simulink library "LIB_UserCommand"  (R2018b)
settings: Solver=VariableStepAuto  StartTime=0.0  StopTime=10.0  RelTol=1e-3
undefined symbols (not defined in the file or in its folder): NCyclePerMinIncrement, pBlowerValveOutletStaticTgtIncrement, pPatientValveInletTgtIncrement, rInhalationPerCycleDefault
libraries: RespiratorCtrlLib x15
settings Model: Creator=BRAUL  LastModifiedBy=BRAUL

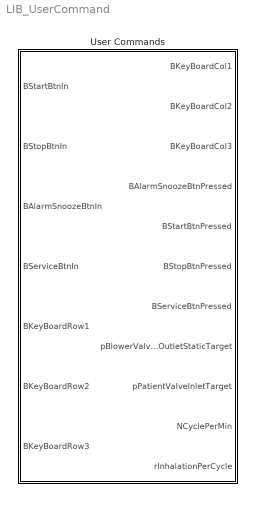
== system LIB_UserCommand ==
  User Commands : Subsystem
      settings: AttributesFormatString=%<ReferenceBlock>

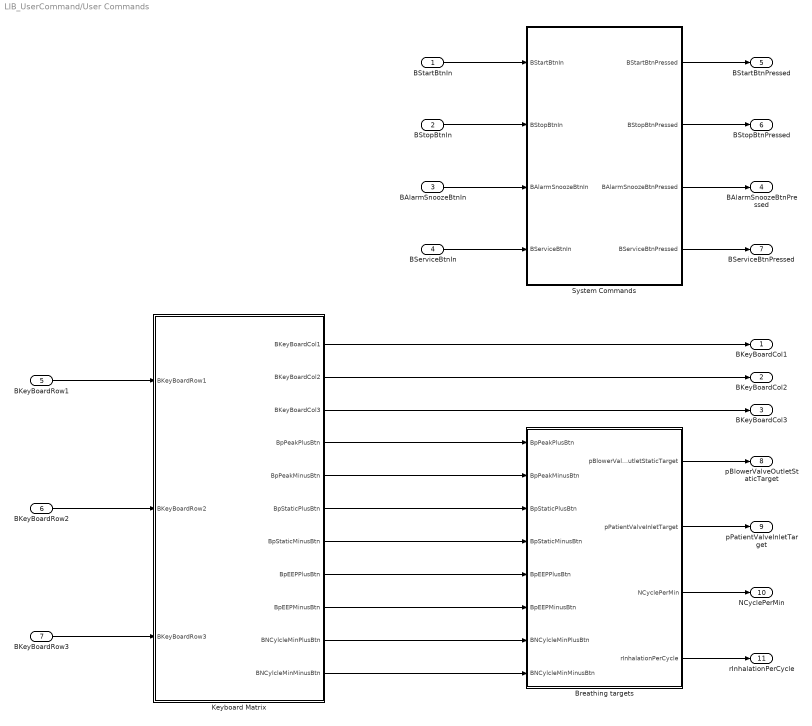
== system LIB_UserCommand/User Commands ==
  BStartBtnIn : Inport  OutDataTypeStr=boolean
  BStopBtnIn : Inport  Port=2  OutDataTypeStr=boolean
  BAlarmSnoozeBtnIn : Inport  Port=3  OutDataTypeStr=boolean
  BServiceBtnIn : Inport  Port=4  OutDataTypeStr=boolean
  BKeyBoardRow1 : Inport  Port=5  OutDataTypeStr=boolean  PortDimensions=1
  BKeyBoardRow2 : Inport  Port=6  OutDataTypeStr=boolean  PortDimensions=1
  BKeyBoardRow3 : Inport  Port=7  OutDataTypeStr=boolean  PortDimensions=1
  Breathing targets : Subsystem
  Keyboard Matrix : Subsystem
  System Commands : Subsystem
  BKeyBoardCol1 : Outport  OutDataTypeStr=boolean  PortDimensions=1
  BKeyBoardCol2 : Outport  Port=2  OutDataTypeStr=boolean  PortDimensions=1
  BKeyBoardCol3 : Outport  Port=3  OutDataTypeStr=boolean  PortDimensions=1
  BAlarmSnoozeBtnPressed : Outport  Port=4  OutDataTypeStr=boolean
  BStartBtnPressed : Outport  Port=5  OutDataTypeStr=boolean
  BStopBtnPressed : Outport  Port=6  OutDataTypeStr=boolean
  BServiceBtnPressed : Outport  Port=7  OutDataTypeStr=boolean
  pBlowerValveOutletStaticTarget : Outport  Port=8
  pPatientValveInletTarget : Outport  Port=9
  NCyclePerMin : Outport  Port=10
  rInhalationPerCycle : Outport  Port=11
  wires:
  BKeyBoardRow3/1 -> Keyboard Matrix/3(BKeyBoardRow3)
  BKeyBoardRow2/1 -> Keyboard Matrix/2(BKeyBoardRow2)
  BKeyBoardRow1/1 -> Keyboard Matrix/1(BKeyBoardRow1)
  Keyboard Matrix/3(BKeyBoardCol3) -> BKeyBoardCol3/1
  Keyboard Matrix/2(BKeyBoardCol2) -> BKeyBoardCol2/1
  Keyboard Matrix/1(BKeyBoardCol1) -> BKeyBoardCol1/1
  Keyboard Matrix/4(BpPeakPlusBtn) -> Breathing targets/1(BpPeakPlusBtn)
  Keyboard Matrix/5(BpPeakMinusBtn) -> Breathing targets/2(BpPeakMinusBtn)
  Keyboard Matrix/6(BpStaticPlusBtn) -> Breathing targets/3(BpStaticPlusBtn)
  Keyboard Matrix/7(BpStaticMinusBtn) -> Breathing targets/4(BpStaticMinusBtn)
  Keyboard Matrix/8(BpEEPPlusBtn) -> Breathing targets/5(BpEEPPlusBtn)
  Keyboard Matrix/9(BpEEPMinusBtn) -> Breathing targets/6(BpEEPMinusBtn)
  Keyboard Matrix/10(BNCylcleMinPlusBtn) -> Breathing targets/7(BNCylcleMinPlusBtn)
  Keyboard Matrix/11(BNCylcleMinMinusBtn) -> Breathing targets/8(BNCylcleMinMinusBtn)
  BStartBtnIn/1 -> System Commands/1(BStartBtnIn)
  BStopBtnIn/1 -> System Commands/2(BStopBtnIn)
  BAlarmSnoozeBtnIn/1 -> System Commands/3(BAlarmSnoozeBtnIn)
  BServiceBtnIn/1 -> System Commands/4(BServiceBtnIn)
  System Commands/1(BStartBtnPressed) -> BStartBtnPressed/1
  System Commands/2(BStopBtnPressed) -> BStopBtnPressed/1
  System Commands/3(BAlarmSnoozeBtnPressed) -> BAlarmSnoozeBtnPressed/1
  System Commands/4(BServiceBtnPressed) -> BServiceBtnPressed/1
  Breathing targets/1(pBlowerValveOutletStaticTarget) -> pBlowerValveOutletStaticTarget/1
  Breathing targets/2(pPatientValveInletTarget) -> pPatientValveInletTarget/1
  Breathing targets/3(NCyclePerMin) -> NCyclePerMin/1
  Breathing targets/4(rInhalationPerCycle) -> rInhalationPerCycle/1

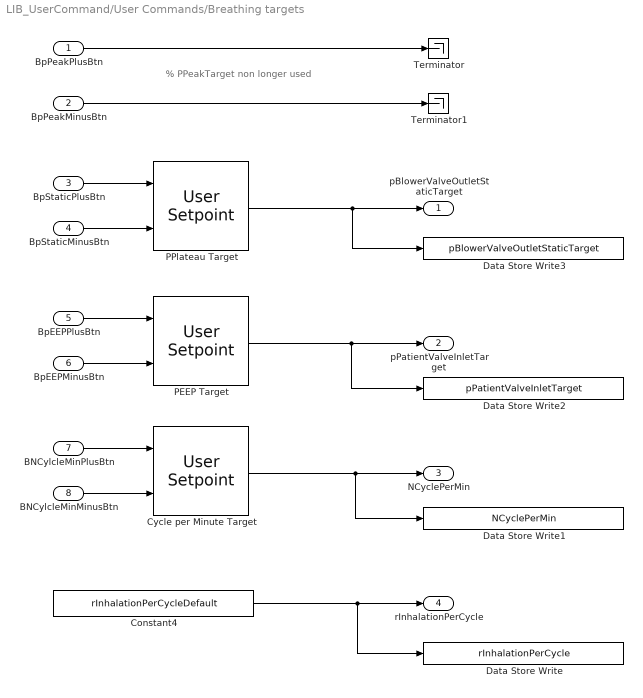
== system LIB_UserCommand/User Commands/Breathing targets ==
  note: % PPeakTarget non longer used
  BpPeakPlusBtn : Inport  OutDataTypeStr=boolean  PortDimensions=1
  BpPeakMinusBtn : Inport  Port=2  OutDataTypeStr=boolean  PortDimensions=1
  BpStaticPlusBtn : Inport  Port=3  OutDataTypeStr=boolean  PortDimensions=1
  BpStaticMinusBtn : Inport  Port=4  OutDataTypeStr=boolean  PortDimensions=1
  BpEEPPlusBtn : Inport  Port=5  OutDataTypeStr=boolean  PortDimensions=1
  BpEEPMinusBtn : Inport  Port=6  OutDataTypeStr=boolean  PortDimensions=1
  BNCylcleMinPlusBtn : Inport  Port=7  OutDataTypeStr=boolean  PortDimensions=1
  BNCylcleMinMinusBtn : Inport  Port=8  OutDataTypeStr=boolean  PortDimensions=1
  Constant4 : Constant  Value=rInhalationPerCycleDefault
  Cycle per Minute Target : RespiratorCtrlLib/Inputs/User Setpoint  DefaultSetPoint=NCyclePerMinDefault  Increment=NCyclePerMinIncrement  Decrement=NCyclePerMinDecrement  MinSetPoint=NCyclePerMinMin  MaxSetPoint=NCyclePerMinMax
  Data Store Write : DataStoreWrite  DataStoreName=rInhalationPerCycle
  Data Store Write1 : DataStoreWrite  DataStoreName=NCyclePerMin
  Data Store Write2 : DataStoreWrite  DataStoreName=pPatientValveInletTarget
  Data Store Write3 : DataStoreWrite  DataStoreName=pBlowerValveOutletStaticTarget
  PEEP Target : RespiratorCtrlLib/Inputs/User Setpoint  DefaultSetPoint=pPatientValveInletTgtDefault  Increment=pPatientValveInletTgtIncrement  Decrement=pPatientValveInletTgtDecrement  MinSetPoint=pPatientValveInletTgtMin  MaxSetPoint=pPatientValveInletTgtMax
  PPlateau Target : RespiratorCtrlLib/Inputs/User Setpoint  DefaultSetPoint=pBlowerValveOutletStaticTgtDefault  Increment=pBlowerValveOutletStaticTgtIncrement  Decrement=pBlowerValveOutletStaticTgtDecrement  MinSetPoint=pBlowerValveOutletStaticTgtMin  MaxSetPoint=pBlowerValveOutletStaticTgtMax
  Terminator : Terminator
  Terminator1 : Terminator
  pBlowerValveOutletStaticTarget : Outport
  pPatientValveInletTarget : Outport  Port=2
  NCyclePerMin : Outport  Port=3
  rInhalationPerCycle : Outport  Port=4
  wires:
  BpPeakMinusBtn/1 -> Terminator1/1
  BpPeakPlusBtn/1 -> Terminator/1
  BNCylcleMinMinusBtn/1 -> Cycle per Minute Target/2
  BNCylcleMinPlusBtn/1 -> Cycle per Minute Target/1
  BpEEPMinusBtn/1 -> PEEP Target/2
  BpEEPPlusBtn/1 -> PEEP Target/1
  BpStaticMinusBtn/1 -> PPlateau Target/2
  BpStaticPlusBtn/1 -> PPlateau Target/1
  Constant4/1 -> rInhalationPerCycle/1, Data Store Write/1
  PEEP Target/1 -> pPatientValveInletTarget/1, Data Store Write2/1
  PPlateau Target/1 -> Data Store Write3/1, pBlowerValveOutletStaticTarget/1
  Cycle per Minute Target/1 -> NCyclePerMin/1, Data Store Write1/1

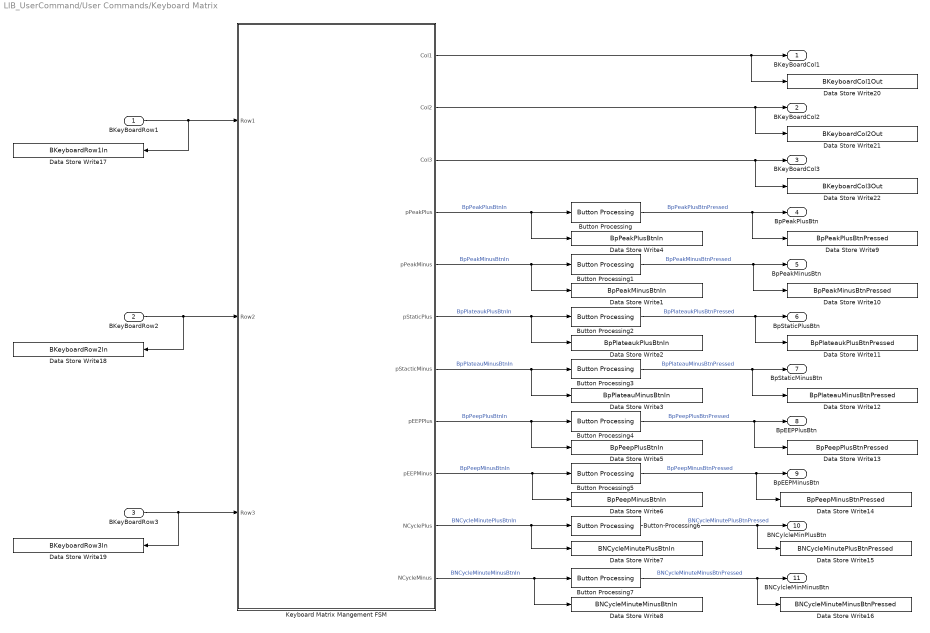
== system LIB_UserCommand/User Commands/Keyboard Matrix ==
  BKeyBoardRow1 : Inport  OutDataTypeStr=boolean  PortDimensions=1
  BKeyBoardRow2 : Inport  Port=2  OutDataTypeStr=boolean  PortDimensions=1
  BKeyBoardRow3 : Inport  Port=3  OutDataTypeStr=boolean  PortDimensions=1
  Button Processing{,1..7} (8 alike) : RespiratorCtrlLib/Inputs/Button Processing  tDebounce=tKeyboardBtnDebounce  tSample=MdlTS
  Data Store Write1 : DataStoreWrite  DataStoreName=BpPeakMinusBtnIn
  Data Store Write10 : DataStoreWrite  DataStoreName=BpPeakMinusBtnPressed
  Data Store Write11 : DataStoreWrite  DataStoreName=BpPlateaukPlusBtnPressed
  Data Store Write12 : DataStoreWrite  DataStoreName=BpPlateauMinusBtnPressed
  Data Store Write13 : DataStoreWrite  DataStoreName=BpPeepPlusBtnPressed
  Data Store Write14 : DataStoreWrite  DataStoreName=BpPeepMinusBtnPressed
  Data Store Write15 : DataStoreWrite  DataStoreName=BNCycleMinutePlusBtnPressed
  Data Store Write16 : DataStoreWrite  DataStoreName=BNCycleMinuteMinusBtnPressed
  Data Store Write17 : DataStoreWrite  DataStoreName=BKeyboardRow1In
  Data Store Write18 : DataStoreWrite  DataStoreName=BKeyboardRow2In
  Data Store Write19 : DataStoreWrite  DataStoreName=BKeyboardRow3In
  Data Store Write2 : DataStoreWrite  DataStoreName=BpPlateaukPlusBtnIn
  Data Store Write20 : DataStoreWrite  DataStoreName=BKeyboardCol1Out
  Data Store Write21 : DataStoreWrite  DataStoreName=BKeyboardCol2Out
  Data Store Write22 : DataStoreWrite  DataStoreName=BKeyboardCol3Out
  Data Store Write3 : DataStoreWrite  DataStoreName=BpPlateauMinusBtnIn
  Data Store Write4 : DataStoreWrite  DataStoreName=BpPeakPlusBtnIn
  Data Store Write5 : DataStoreWrite  DataStoreName=BpPeepPlusBtnIn
  Data Store Write6 : DataStoreWrite  DataStoreName=BpPeepMinusBtnIn
  Data Store Write7 : DataStoreWrite  DataStoreName=BNCycleMinutePlusBtnIn
  Data Store Write8 : DataStoreWrite  DataStoreName=BNCycleMinuteMinusBtnIn
  Data Store Write9 : DataStoreWrite  DataStoreName=BpPeakPlusBtnPressed
  Keyboard Matrix Mangement FSM : Stateflow chart  TreatAsAtomicUnit=on
  BKeyBoardCol1 : Outport  OutDataTypeStr=boolean  PortDimensions=1
  BKeyBoardCol2 : Outport  Port=2  OutDataTypeStr=boolean  PortDimensions=1
  BKeyBoardCol3 : Outport  Port=3  OutDataTypeStr=boolean  PortDimensions=1
  BpPeakPlusBtn : Outport  Port=4  OutDataTypeStr=boolean  PortDimensions=1
  BpPeakMinusBtn : Outport  Port=5  OutDataTypeStr=boolean  PortDimensions=1
  BpStaticPlusBtn : Outport  Port=6  OutDataTypeStr=boolean  PortDimensions=1
  BpStaticMinusBtn : Outport  Port=7  OutDataTypeStr=boolean  PortDimensions=1
  BpEEPPlusBtn : Outport  Port=8  OutDataTypeStr=boolean  PortDimensions=1
  BpEEPMinusBtn : Outport  Port=9  OutDataTypeStr=boolean  PortDimensions=1
  BNCylcleMinPlusBtn : Outport  Port=10  OutDataTypeStr=boolean  PortDimensions=1
  BNCylcleMinMinusBtn : Outport  Port=11  OutDataTypeStr=boolean  PortDimensions=1
  wires:
  Button Processing7/1 -> BNCylcleMinMinusBtn/1, Data Store Write16/1  "BNCycleMinuteMinusBtnPressed"
  Button Processing6/1 -> BNCylcleMinPlusBtn/1, Data Store Write15/1  "BNCycleMinutePlusBtnPressed"
  Button Processing5/1 -> BpEEPMinusBtn/1, Data Store Write14/1  "BpPeepMinusBtnPressed"
  Button Processing4/1 -> BpEEPPlusBtn/1, Data Store Write13/1  "BpPeepPlusBtnPressed"
  Button Processing3/1 -> BpStaticMinusBtn/1, Data Store Write12/1  "BpPlateauMinusBtnPressed"
  Button Processing2/1 -> BpStaticPlusBtn/1, Data Store Write11/1  "BpPlateaukPlusBtnPressed"
  Button Processing1/1 -> BpPeakMinusBtn/1, Data Store Write10/1  "BpPeakMinusBtnPressed"
  Button Processing/1 -> BpPeakPlusBtn/1, Data Store Write9/1  "BpPeakPlusBtnPressed"
  Keyboard Matrix Mangement FSM/10(NCyclePlus) -> Button Processing6/1, Data Store Write7/1  "BNCycleMinutePlusBtnIn"
  Keyboard Matrix Mangement FSM/11(NCycleMinus) -> Button Processing7/1, Data Store Write8/1  "BNCycleMinuteMinusBtnIn"
  Keyboard Matrix Mangement FSM/9(pEEPMinus) -> Button Processing5/1, Data Store Write6/1  "BpPeepMinusBtnIn"
  Keyboard Matrix Mangement FSM/8(pEEPPlus) -> Button Processing4/1, Data Store Write5/1  "BpPeepPlusBtnIn"
  Keyboard Matrix Mangement FSM/7(pStacticMinus) -> Button Processing3/1, Data Store Write3/1  "BpPlateauMinusBtnIn"
  Keyboard Matrix Mangement FSM/6(pStaticPlus) -> Button Processing2/1, Data Store Write2/1  "BpPlateaukPlusBtnIn"
  Keyboard Matrix Mangement FSM/5(pPeakMinus) -> Button Processing1/1, Data Store Write1/1  "BpPeakMinusBtnIn"
  Keyboard Matrix Mangement FSM/4(pPeakPlus) -> Button Processing/1, Data Store Write4/1  "BpPeakPlusBtnIn"
  BKeyBoardRow1/1 -> Keyboard Matrix Mangement FSM/1(Row1), Data Store Write17/1
  BKeyBoardRow2/1 -> Keyboard Matrix Mangement FSM/2(Row2), Data Store Write18/1
  BKeyBoardRow3/1 -> Keyboard Matrix Mangement FSM/3(Row3), Data Store Write19/1
  Keyboard Matrix Mangement FSM/3(Col3) -> BKeyBoardCol3/1, Data Store Write22/1
  Keyboard Matrix Mangement FSM/2(Col2) -> BKeyBoardCol2/1, Data Store Write21/1
  Keyboard Matrix Mangement FSM/1(Col1) -> BKeyBoardCol1/1, Data Store Write20/1

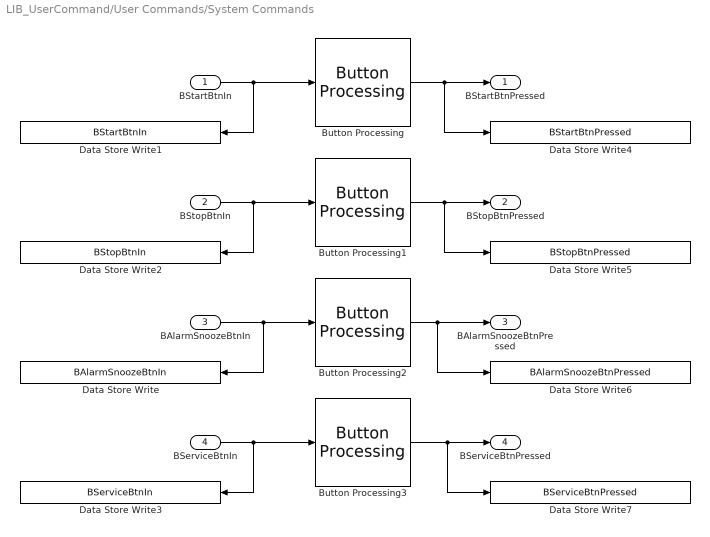
== system LIB_UserCommand/User Commands/System Commands ==
  BStartBtnIn : Inport  OutDataTypeStr=boolean
  BStopBtnIn : Inport  Port=2  OutDataTypeStr=boolean
  BAlarmSnoozeBtnIn : Inport  Port=3  OutDataTypeStr=boolean
  BServiceBtnIn : Inport  Port=4  OutDataTypeStr=boolean
  Button Processing{,1..3} (4 alike) : RespiratorCtrlLib/Inputs/Button Processing  tDebounce=tSystemBtnDebounce  tSample=MdlTS
  Data Store Write : DataStoreWrite  DataStoreName=BAlarmSnoozeBtnIn
  Data Store Write1 : DataStoreWrite  DataStoreName=BStartBtnIn
  Data Store Write2 : DataStoreWrite  DataStoreName=BStopBtnIn
  Data Store Write3 : DataStoreWrite  DataStoreName=BServiceBtnIn
  Data Store Write4 : DataStoreWrite  DataStoreName=BStartBtnPressed
  Data Store Write5 : DataStoreWrite  DataStoreName=BStopBtnPressed
  Data Store Write6 : DataStoreWrite  DataStoreName=BAlarmSnoozeBtnPressed
  Data Store Write7 : DataStoreWrite  DataStoreName=BServiceBtnPressed
  BStartBtnPressed : Outport  OutDataTypeStr=boolean
  BStopBtnPressed : Outport  Port=2  OutDataTypeStr=boolean
  BAlarmSnoozeBtnPressed : Outport  Port=3  OutDataTypeStr=boolean
  BServiceBtnPressed : Outport  Port=4  OutDataTypeStr=boolean
  wires:
  Button Processing/1 -> Data Store Write4/1, BStartBtnPressed/1
  BStartBtnIn/1 -> Data Store Write1/1, Button Processing/1
  BStopBtnIn/1 -> Data Store Write2/1, Button Processing1/1
  BAlarmSnoozeBtnIn/1 -> Data Store Write/1, Button Processing2/1
  BServiceBtnIn/1 -> Data Store Write3/1, Button Processing3/1
  Button Processing1/1 -> Data Store Write5/1, BStopBtnPressed/1
  Button Processing2/1 -> Data Store Write6/1, BAlarmSnoozeBtnPressed/1
  Button Processing3/1 -> Data Store Write7/1, BServiceBtnPressed/1

== stateflow chart LIB_UserCommand/User Commands/Keyboard Matrix/Keyboard Matrix Mangement FSM ==
  state Init
    entry:
    Col1 = true;
    Col2 = false;
    Col3 = false;
  state READ_COL_1
    entry:
    Col1 = false;
    Col2 = true;
    Col3 = false;
    pPeakPlus = Row1;
    pPeakMinus  = Row2;
    pStaticPlus  = Row3;
  state READ_COL_3
    entry:
    Col1 = true;
    Col2 = false;
    Col3 = false;
    NCyclePlus = Row1;
    NCycleMinus  = Row2;
  state READ_COL_2
    entry:
    Col1 = false;
    Col2 = false;
    Col3 = true;
    pStacticMinus = Row1;
    pEEPPlus  = Row2;
    pEEPMinus  = Row3;
  (default) -> Init
  Init -> READ_COL_1
  READ_COL_3 -> READ_COL_1
  READ_COL_1 -> READ_COL_2
  READ_COL_2 -> READ_COL_3
  data: Row1 input boolean; Row2 input boolean; Row3 input boolean; Col1 output boolean =false; Col2 output boolean =false; Col3 output boolean =false; pPeakPlus output boolean =false; pPeakMinus output boolean =false; pStaticPlus output boolean =false; pStacticMinus output boolean =false; pEEPPlus output boolean =false; pEEPMinus output boolean =false; NCyclePlus output boolean =false; NCycleMinus output boolean =false
